simulink model "input_increasing_scheme"  (R2017a)
settings: Solver=VariableStepAuto  StartTime=0.0  StopTime=0.013  MaxStep=1e-4  RelTol=1e-4  EnableMultiTasking=on
libraries: powerlib x17, powerlib_meascontrol x1
Description:
  | Copyright 2008-2017 The MathWorks, Inc.
settings Model: Creator=MathWorks  LastModifiedBy=re
settings SolverCC: SolverResetMethod=Robust
settings DataIOCC: ReturnWorkspaceOutputs=on
settings OptimizationCC: LifeSpan=inf
settings DebuggingCC: ReadBeforeWriteMsg=DisableAll  WriteAfterWriteMsg=DisableAll  WriteAfterReadMsg=DisableAll  MultiTaskDSMMsg=none  SFUnexpectedBacktrackingDiag=warning  SFNoUnconditionalDefaultTransitionDiag=warning  SFExecutionAtInitializationDiag=none
settings ModelReferenceCC: UpdateModelReferenceTargets=IfOutOfDate
settings SFSimCC: SFSimEcho=off
settings GRTTargetCC: TargetLangStandard=C89/C90 (ANSI)  GeneratePreprocessorConditionals=Disable all
settings ConfigComp: CovMetricSettings=dw  CovHtmlReporting=on  CovSaveCumulativeToWorkspaceVar=on  CovSaveSingleToWorkspaceVar=on  CovExternalEMLEnable=off

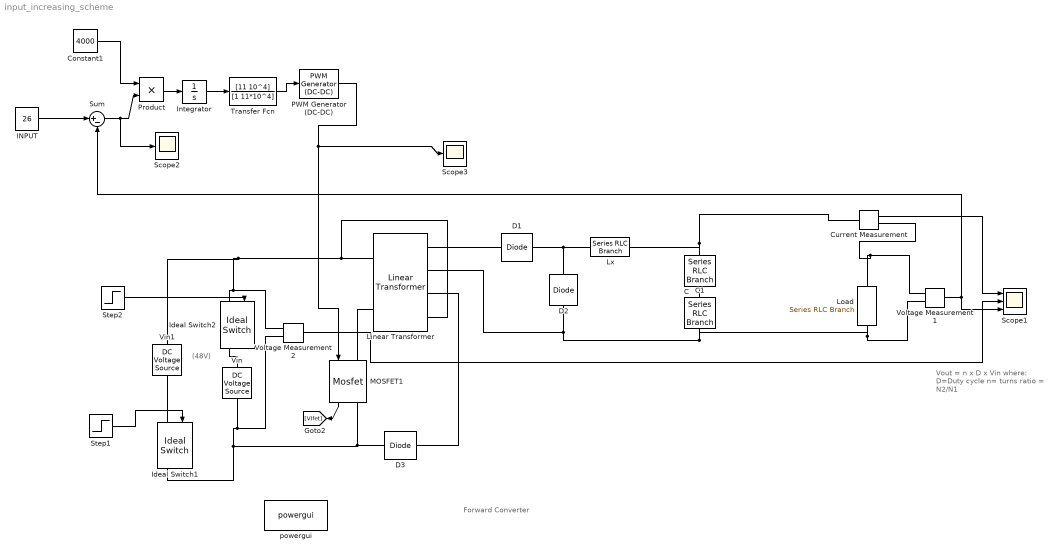
== system input_increasing_scheme ==
  note: Vout = n x D x Vin
      | where: D=Duty cycle
      | n= turns ratio = N2/N1
  note: (48V)
  note: Forward Converter
  C : powerlib/Elements/Series RLC Branch  LConnTagsString=__new0  RConnTagsString=__new0  BranchType=RC  Resistance=0.00166  Inductance=200e-6  SetiL0=off  InitialCurrent=0  Capacitance=30e-6  Setx0=off  InitialVoltage=0  Measurements=None
  C1 : powerlib/Elements/Series RLC Branch  LConnTagsString=__new0  RConnTagsString=__new0  BranchType=RC  Resistance=1.2  Inductance=200e-6  SetiL0=off  InitialCurrent=0  Capacitance=100e-6  Setx0=off  InitialVoltage=0  Measurements=None
  Constant1 : Constant  Value=4000
  Current Measurement : powerlib/Measurements/Current Measurement  PhasorSimulation=off  OutputType=Complex  PSBequivalent=0
  D1 : powerlib/Power Electronics/Diode  Ron=1e-3  Lon=0  Vf=0.7  IC=0  UseSnubber=off  Rs=inf  Cs=0  Measurements=off
  D2 : powerlib/Power Electronics/Diode  Ron=1e-3  Lon=0  Vf=0.7  IC=0  UseSnubber=off  Rs=inf  Cs=0  Measurements=off
  D3 : powerlib/Power Electronics/Diode  Ron=1e-3  Lon=0  Vf=0.7  IC=0  UseSnubber=off  Rs=inf  Cs=0  Measurements=off
  INPUT : Constant  Value=26
  Ideal Switch1 : powerlib/Power Electronics/Ideal Switch  Ron=0.001  Lon=0  IC=0  Rs=1e5  Cs=inf  Measurements=on
  Ideal Switch2 : powerlib/Power Electronics/Ideal Switch  Ron=0.001  Lon=0  IC=0  Rs=1e5  Cs=inf  Measurements=on
  Integrator : Integrator
  Linear Transformer : powerlib/Elements/Linear Transformer  UNITS=SI  NominalPower=[ 25 100e3 ]  winding1=[48 0 0]  winding2=[74 0 0]  ThreeWindings=on  winding3=[48 0 0]  RmLm=[inf 10e-3]  Measurements=Magnetization current  DataType=on
  Load : powerlib/Elements/Series RLC Branch  LConnTagsString=__new0  RConnTagsString=__new0  BranchType=R  Resistance=7  Inductance=200e-6  SetiL0=off  InitialCurrent=0  Capacitance=400e-6  Setx0=off  InitialVoltage=0  Measurements=Branch current
  Lx : powerlib/Elements/Series RLC Branch  LConnTagsString=__new0  RConnTagsString=__new0  BranchType=RL  Resistance=0.085  Inductance=94e-6  SetiL0=off  InitialCurrent=0  Capacitance=400e-6  Setx0=off  InitialVoltage=0  Measurements=Branch current
  MOSFET1 : powerlib/Power Electronics/Mosfet  Ron=1e-3  Lon=0  Rd=1e-3  Vfd=0  IC=0  Rs=1e6  Cs=inf  Measurements=on
  PWM Generator (DC-DC) : powerlib_meascontrol/Pulse & Signal Generators/PWM Generator (DC-DC)  Fsw=200000  Ts=0
  Product : Product
  Scope1 : Scope  NumInputPorts=3
  Scope2 : Scope
  Scope3 : Scope
  Step1 : Step  Time=0.007  SampleTime=0
  Step2 : Step  Time=0.007  Before=1  After=0  SampleTime=0
  Sum : Sum  Inputs=|+-
  Transfer Fcn : TransferFcn  Numerator=[11 10^4]  Denominator=[1 11*10^4]
  Vin : powerlib/Electrical Sources/DC Voltage Source  Amplitude=48  Measurements=None
  Vin1 : powerlib/Electrical Sources/DC Voltage Source  Amplitude=52  Measurements=None
  Voltage Measurement1 : powerlib/Measurements/Voltage Measurement  PhasorSimulation=off  OutputType=Complex  PSBequivalent=0
  Voltage Measurement2 : powerlib/Measurements/Voltage Measurement  PhasorSimulation=off  OutputType=Complex  PSBequivalent=0
  powergui : powerlib/powergui  Priority=1  SimulationMode=Continuous  SampleTime=50e-6  frequency=60  Iterations=50  frequencyindice=0  Pbase=100e6  ErrMax=1e-4  UnitsV=kV  UnitsW=MW  buscounter=0  FunctionMessages=off  echomessages=off  EnableUseOfTLC=off  CurrentSourceSwitches=off  DisableSnubberDevices=off  DisableRonSwitches=off  DisableVfSwitches=off  DisplayEquations=off  SolverType=Tustin/Backward Euler (TBE)  Interpol=off  ExternalGateDelay=off  methode=off  Ts=100  x0status=blocks  SPID=on  SwTol=0  HookPort=off  RestoreLinks=warning  ResistiveCurrentMeasurement=off  Frange=[0:2:500]  Ylog=off  Xlog=on  ShowGrid=off  save=off  variable=ZData  structure=0  ZoomFFT=off  StartTime=0.0  cycles=1  DisplayStyle=1  fundamental=60  FreqAxis=off  MaxFrequency=1000  frequencyindicesteady=1  RmsSteady=1  display=off
  wires:
  MOSFET1/1 -> [VIfet]
  Integrator/1 -> Transfer Fcn/1
  Transfer Fcn/1 -> PWM Generator (DC-DC)/1
  Voltage Measurement1/1 -> Sum/2, Scope1/3
  Product/1 -> Integrator/1
  Constant1/1 -> Product/1
  Sum/1 -> Scope2/1, Product/2
  PWM Generator (DC-DC)/1 -> Scope3/1, MOSFET1/1
  INPUT/1 -> Sum/1
  Voltage Measurement2/1 -> Scope1/2
  Current Measurement/1 -> Scope1/1
  Step1/1 -> Ideal Switch1/1
  Step2/1 -> Ideal Switch2/1
  connections:
  Current Measurement/LConn1 -- Lx/RConn1 -- C/LConn1
  D2/LConn1 -- Voltage Measurement1/LConn2 -- Load/RConn1 -- C1/RConn1 -- Linear Transformer/RConn2
  Linear Transformer/LConn2 -- MOSFET1/LConn1
  D3/LConn1 -- Vin/LConn1 -- Voltage Measurement2/LConn2 -- Ideal Switch1/RConn1 -- MOSFET1/RConn1
  Linear Transformer/RConn4 -- Voltage Measurement2/LConn1 -- Ideal Switch2/LConn1 -- Vin1/RConn1 -- Linear Transformer/LConn1
  D1/LConn1 -- Linear Transformer/RConn1
  D2/RConn1 -- D1/RConn1 -- Lx/LConn1
  D3/RConn1 -- Linear Transformer/RConn3
  Load/LConn1 -- Current Measurement/RConn1 -- Voltage Measurement1/LConn1
  C/RConn1 -- C1/LConn1
  Vin1/LConn1 -- Ideal Switch1/LConn1
  Vin/RConn1 -- Ideal Switch2/RConn1
